simulink library "INT_InjCrv_PiI"  (R2016b)
settings: Solver=VariableStepAuto  StartTime=0.0  StopTime=10.0  RelTol=1e-3
settings Model: Creator=Administrator  LastModifiedBy=Administrator

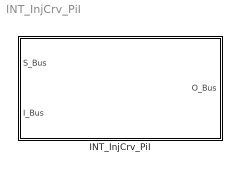
== system INT_InjCrv_PiI ==
  INT_InjCrv_PiI : Subsystem

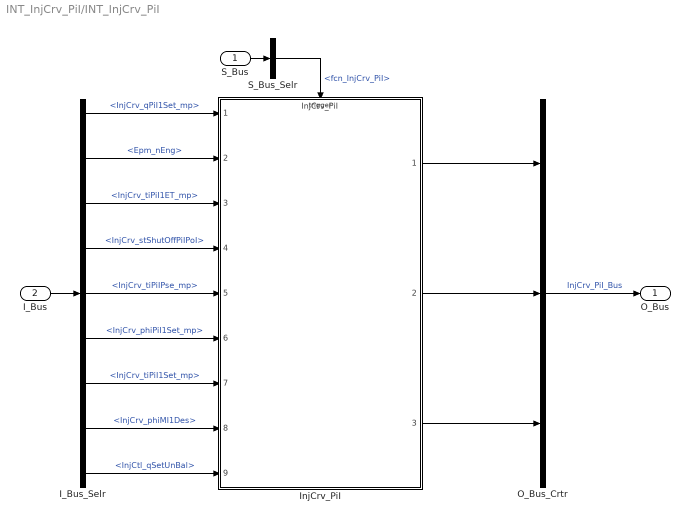
== system INT_InjCrv_PiI/INT_InjCrv_PiI ==
  S_Bus : Inport
  I_Bus : Inport  Port=2
  I_Bus_Selr : BusSelector  OutputSignals=InjCrv_qPiI1Set_mp,Epm_nEng,InjCrv_tiPiI1ET_mp,InjCrv_stShutOffPiIPoI,InjCrv_tiPiIPse_mp,InjCrv_phiPiI1Set_mp,InjCrv_tiPiI1Set_mp,InjCrv_phiMI1Des,InjCtl_qSetUnBal
  InjCrv_PiI : ModelReference  ModelNameDialog=InjCrv_PiI  SimulationMode=Normal  ModelReferenceVersion=1.25  TriggerPortName=function  TriggerPortTriggerType=function-call  TriggerPortStatesWhenEnabling=held
  O_Bus_Crtr : BusCreator  Inputs=3
  S_Bus_Selr : BusSelector  OutputSignals=fcn_InjCrv_PiI
  O_Bus : Outport
  wires:
  S_Bus_Selr/1 -> InjCrv_PiI/Trigger  "<fcn_InjCrv_PiI>"
  S_Bus/1 -> S_Bus_Selr/1
  I_Bus/1 -> I_Bus_Selr/1
  I_Bus_Selr/1 -> InjCrv_PiI/1  "<InjCrv_qPiI1Set_mp>"
  I_Bus_Selr/2 -> InjCrv_PiI/2  "<Epm_nEng>"
  I_Bus_Selr/3 -> InjCrv_PiI/3  "<InjCrv_tiPiI1ET_mp>"
  I_Bus_Selr/4 -> InjCrv_PiI/4  "<InjCrv_stShutOffPiIPoI>"
  I_Bus_Selr/5 -> InjCrv_PiI/5  "<InjCrv_tiPiIPse_mp>"
  I_Bus_Selr/6 -> InjCrv_PiI/6  "<InjCrv_phiPiI1Set_mp>"
  I_Bus_Selr/7 -> InjCrv_PiI/7  "<InjCrv_tiPiI1Set_mp>"
  I_Bus_Selr/8 -> InjCrv_PiI/8  "<InjCrv_phiMI1Des>"
  I_Bus_Selr/9 -> InjCrv_PiI/9  "<InjCtl_qSetUnBal>"
  O_Bus_Crtr/1 -> O_Bus/1  "InjCrv_PiI_Bus"
  InjCrv_PiI/1 -> O_Bus_Crtr/1
  InjCrv_PiI/2 -> O_Bus_Crtr/2
  InjCrv_PiI/3 -> O_Bus_Crtr/3
